simulink model "PitchPlunge"  (R2015a)
settings: Solver=ode3  StartTime=0.0  StopTime=T  FixedStep=dt  RelTol=1e-3
values from neighbouring files (symbols this model uses):
  dt = 0.01    [Main.m]
  gamma = 0.5    [Main.m]
  U0 = 15    [Main.m]
  useNonlinear = 0    [Main.m]
undefined symbols (not defined in the file or in its folder): C, D, E, F, initialTurbulence, ka, ka1, ka2, ka3, ka4, kh, Light, M, MIL, Q, R, stateFilterGamma, turbulenceFactor, turbulenceSeed, x0, xd0
libraries: aerolibwind2 x1
settings Model: Creator=hildobijl  LastModifiedBy=Hildo
settings DataIOCC: SignalLoggingSaveFormat=ModelDataLogs
settings OptimizationCC: ExpressionDepthLimit=2147483647
settings DebuggingCC: SolverPrmCheckMsg=warning  FcnCallInpInsideContextMsg=EnableAllAsWarning  StateNameClashWarn=warning
settings GRTTargetCC: CombineOutputUpdateFcns=off  GRTInterface=on

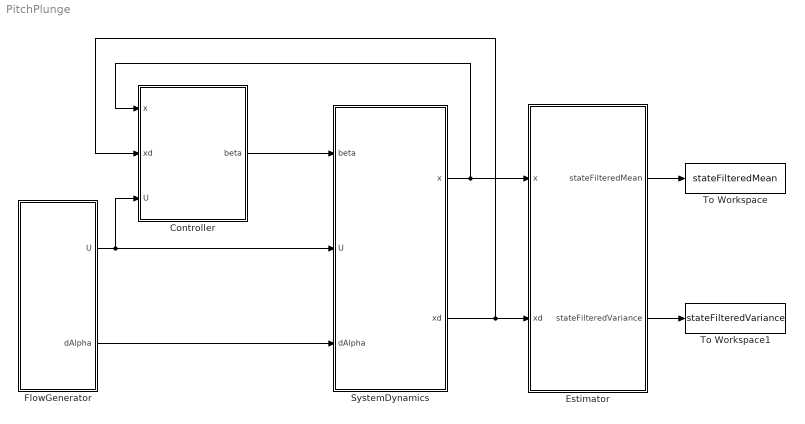
== system PitchPlunge ==
  Controller : Subsystem
  Estimator : Subsystem
  FlowGenerator : Subsystem
  SystemDynamics : Subsystem
  To Workspace : ToWorkspace  VariableName=stateFilteredMean  SampleTime=-1
  To Workspace1 : ToWorkspace  VariableName=stateFilteredVariance  SampleTime=-1
  wires:
  FlowGenerator/1(U) -> Controller/3(U), SystemDynamics/2(U)
  Controller/1(beta) -> SystemDynamics/1(beta)
  SystemDynamics/1(x) -> Controller/1(x), Estimator/1(x)
  SystemDynamics/2(xd) -> Controller/2(xd), Estimator/2(xd)
  FlowGenerator/2(dAlpha) -> SystemDynamics/3(dAlpha)
  Estimator/1(stateFilteredMean) -> To Workspace/1
  Estimator/2(stateFilteredVariance) -> To Workspace1/1

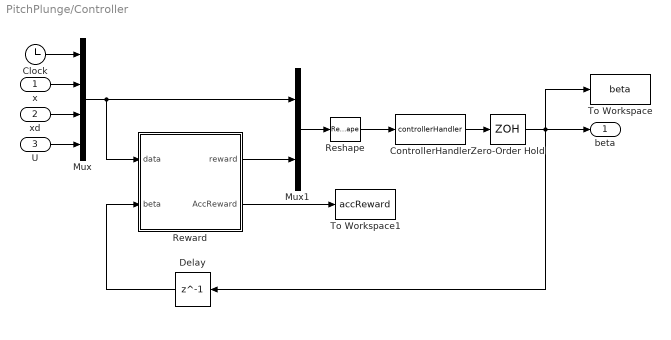
== system PitchPlunge/Controller ==
  x : Inport
  xd : Inport  Port=2
  U : Inport  Port=3
  Clock : Clock
  ControllerHandler : MATLABFcn  MATLABFcn=controllerHandler  SampleTime=dt
  Delay : Delay  DelayLength=1  InitialCondition=0
  Mux : Mux  Inputs=[1,2,2,1]
  Mux1 : Mux  Inputs=[6,1]
  Reshape : Reshape
  Reward : Subsystem
  To Workspace : ToWorkspace  VariableName=beta  SampleTime=-1
  To Workspace1 : ToWorkspace  VariableName=accReward  SampleTime=-1
  Zero-Order Hold : ZeroOrderHold  SampleTime=dt
  beta : Outport
  wires:
  Mux/1 -> Reward/1(data), Mux1/1
  Clock/1 -> Mux/1
  x/1 -> Mux/2
  xd/1 -> Mux/3
  U/1 -> Mux/4
  ControllerHandler/1 -> Zero-Order Hold/1
  Reward/1(reward) -> Mux1/2
  Mux1/1 -> Reshape/1
  Reshape/1 -> ControllerHandler/1
  Zero-Order Hold/1 -> Delay/1, beta/1, To Workspace/1
  Reward/2(AccReward) -> To Workspace1/1
  Delay/1 -> Reward/2(beta)

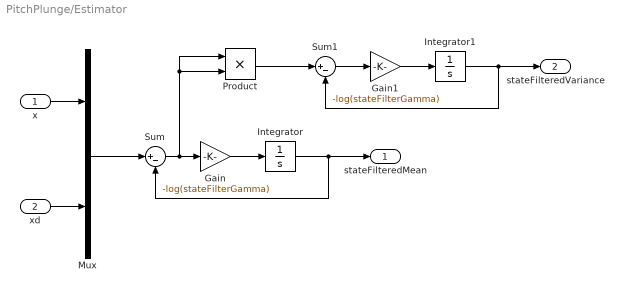
== system PitchPlunge/Estimator ==
  x : Inport
  xd : Inport  Port=2
  Gain : Gain  Gain=-log(stateFilterGamma)
  Gain1 : Gain  Gain=-log(stateFilterGamma)
  Integrator : Integrator  InitialCondition=[x0,xd0]'
  Integrator1 : Integrator
  Mux : Mux  Inputs=[2,2]
  Product : Product
  Sum : Sum  Inputs=|+-
  Sum1 : Sum  Inputs=|+-
  stateFilteredMean : Outport
  stateFilteredVariance : Outport  Port=2
  wires:
  x/1 -> Mux/1
  xd/1 -> Mux/2
  Mux/1 -> Sum/1
  Sum/1 -> Product/1, Product/2, Gain/1
  Integrator/1 -> Sum/2, stateFilteredMean/1
  Gain/1 -> Integrator/1
  Integrator1/1 -> Sum1/2, stateFilteredVariance/1
  Gain1/1 -> Integrator1/1
  Sum1/1 -> Gain1/1
  Product/1 -> Sum1/1

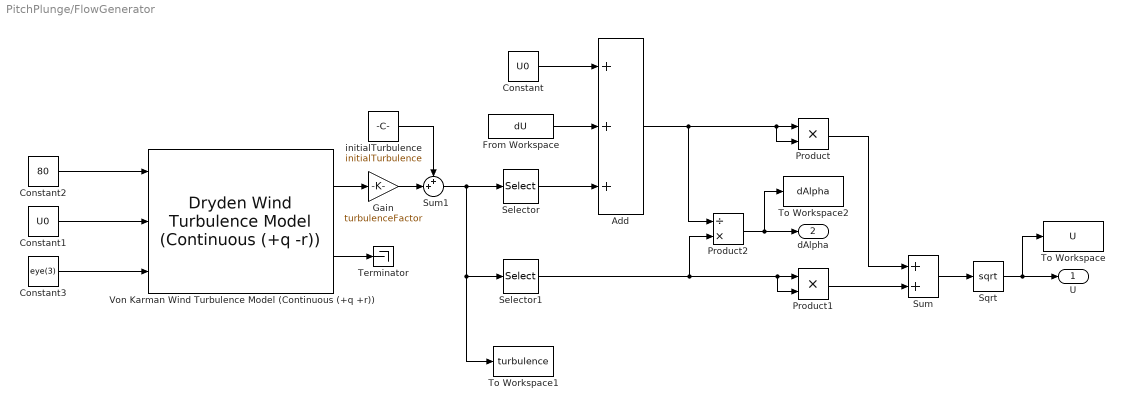
== system PitchPlunge/FlowGenerator ==
  Add : Sum  Inputs=+++
  Constant : Constant  Value=U0
  Constant1 : Constant  Value=U0
  Constant2 : Constant  Value=80
  Constant3 : Constant  Value=eye(3)
  From Workspace : FromWorkspace  VariableName=dU  SampleTime=dt  OutputAfterFinalValue=Holding final value
  Gain : Gain  Gain=turbulenceFactor
  Product : Product
  Product1 : Product
  Product2 : Product  Inputs=/*
  Selector : Selector  InputPortWidth=3  Indices=[1]
  Selector1 : Selector  InputPortWidth=3  Indices=[2]
  Sqrt : Sqrt  SaturateOnIntegerOverflow=on
  Sum : Sum
  Sum1 : Sum  Inputs=++|
  Terminator : Terminator
  To Workspace : ToWorkspace  VariableName=U  SampleTime=-1
  To Workspace1 : ToWorkspace  VariableName=turbulence  SampleTime=-1
  To Workspace2 : ToWorkspace  VariableName=dAlpha  SampleTime=-1
  Von Karman Wind Turbulence Model (Continuous (+q +r)) : aerolibwind2/Dryden Wind Turbulence Model  (Continuous (+q -r))  units=Metric (MKS)  spec=MIL-F-8785C  model=Continuous Von Karman (+q +r)  W20=U0  Wdeg=0  TurbProb=10^-2 - Light  L_high=762  Wingspan=10  ts=dt  Seed=turbulenceSeed  T_on=on
  initialTurbulence : Constant  Value=initialTurbulence
  U : Outport
  dAlpha : Outport  Port=2
  wires:
  Constant/1 -> Add/1
  From Workspace/1 -> Add/2
  Constant2/1 -> Von Karman Wind Turbulence Model (Continuous (+q +r))/1
  Constant1/1 -> Von Karman Wind Turbulence Model (Continuous (+q +r))/2
  Constant3/1 -> Von Karman Wind Turbulence Model (Continuous (+q +r))/3
  Von Karman Wind Turbulence Model (Continuous (+q +r))/2 -> Terminator/1
  Von Karman Wind Turbulence Model (Continuous (+q +r))/1 -> Gain/1
  Selector/1 -> Add/3
  Add/1 -> Product2/1, Product/2, Product/1
  Selector1/1 -> Product2/2, Product1/2, Product1/1
  Product/1 -> Sum/1
  Product1/1 -> Sum/2
  Sum/1 -> Sqrt/1
  Sqrt/1 -> U/1, To Workspace/1
  Product2/1 -> To Workspace2/1, dAlpha/1
  initialTurbulence/1 -> Sum1/1
  Gain/1 -> Sum1/2
  Sum1/1 -> To Workspace1/1, Selector1/1, Selector/1

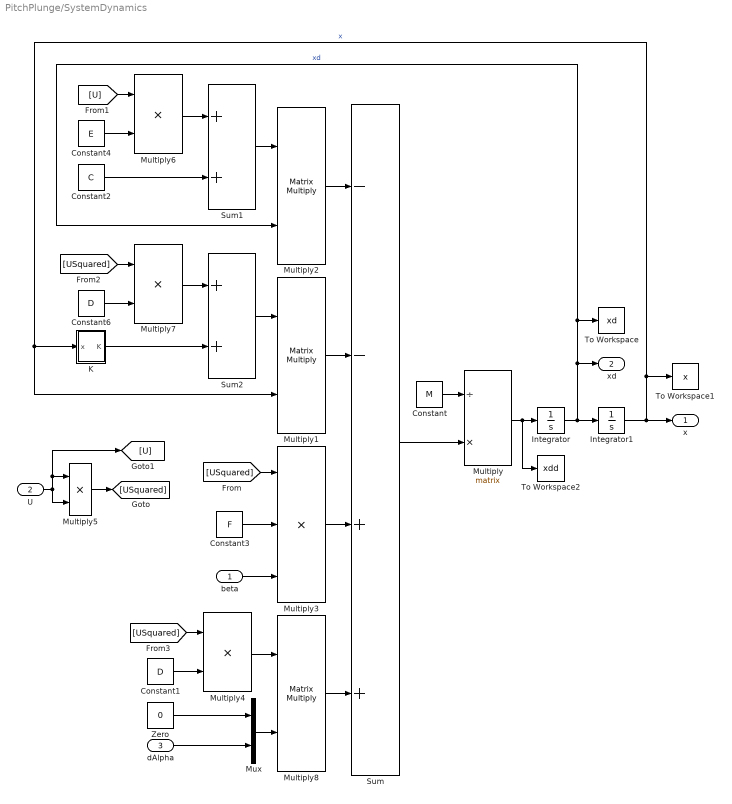
== system PitchPlunge/SystemDynamics ==
  beta : Inport
  U : Inport  Port=2
  dAlpha : Inport  Port=3
  Constant : Constant  Value=M
  Constant1 : Constant  Value=D
  Constant2 : Constant  Value=C
  Constant3 : Constant  Value=F
  Constant4 : Constant  Value=E
  Constant6 : Constant  Value=D
  Integrator : Integrator  InitialCondition=xd0
  Integrator1 : Integrator  InitialCondition=x0
  K : Subsystem
  Multiply : Product  Inputs=/*  Multiplication=Matrix(*)
  Multiply1 : Product  Inputs=**  Multiplication=Matrix(*)
  Multiply2 : Product  Inputs=**  Multiplication=Matrix(*)
  Multiply3 : Product  Inputs=***
  Multiply{4..7} (4 alike) : Product  Inputs=**
  Multiply8 : Product  Inputs=**  Multiplication=Matrix(*)
  Mux : Mux  Inputs=2
  Sum : Sum  Inputs=--++
  Sum1 : Sum
  Sum2 : Sum
  To Workspace : ToWorkspace  VariableName=xd  SampleTime=-1
  To Workspace1 : ToWorkspace  VariableName=x  SampleTime=-1
  To Workspace2 : ToWorkspace  VariableName=xdd  SampleTime=-1
  Zero : Constant  Value=0
  x : Outport
  xd : Outport  Port=2
  wires:
  Integrator/1 -> Integrator1/1, xd/1, To Workspace/1, Multiply2/2  "xd"
  Integrator1/1 -> x/1, To Workspace1/1, Multiply1/2, K/1(x)  "x"
  Multiply/1 -> To Workspace2/1, Integrator/1
  Constant/1 -> Multiply/1
  Sum/1 -> Multiply/2
  Multiply3/1 -> Sum/3
  Multiply2/1 -> Sum/1
  U/1 -> Multiply5/2, Multiply5/1, [U]
  Multiply5/1 -> [USquared]
  [U] -> Multiply6/1
  Constant4/1 -> Multiply6/2
  Multiply6/1 -> Sum1/1
  Constant2/1 -> Sum1/2
  Sum1/1 -> Multiply2/1
  [USquared] -> Multiply7/1
  Constant6/1 -> Multiply7/2
  Multiply7/1 -> Sum2/1
  Sum2/1 -> Multiply1/1
  Multiply1/1 -> Sum/2
  [USquared] -> Multiply3/1
  Constant3/1 -> Multiply3/2
  beta/1 -> Multiply3/3
  K/1(K) -> Sum2/2
  [USquared] -> Multiply4/1
  Constant1/1 -> Multiply4/2
  Zero/1 -> Mux/1
  dAlpha/1 -> Mux/2
  Multiply8/1 -> Sum/4
  Multiply4/1 -> Multiply8/1
  Mux/1 -> Multiply8/2

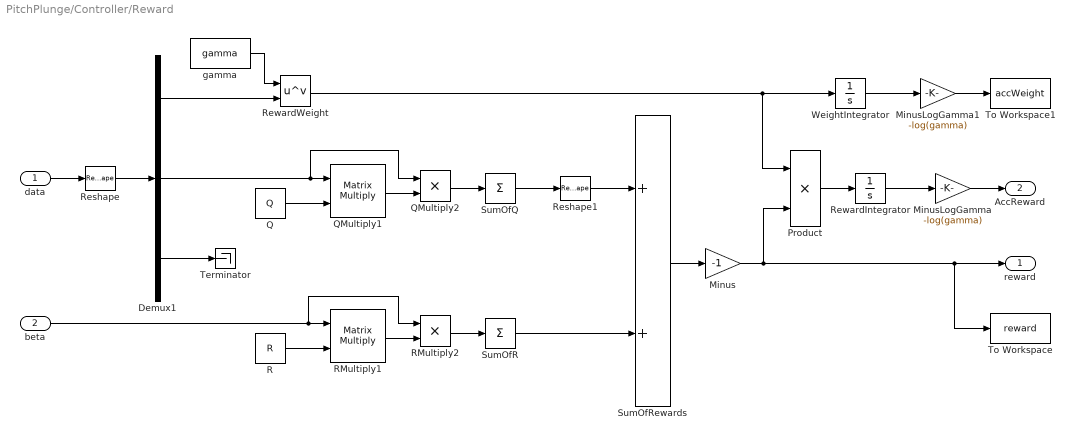
== system PitchPlunge/Controller/Reward ==
  data : Inport
  beta : Inport  Port=2
  Demux1 : Demux  Outputs=[1,4,1]
  Minus : Gain  Gain=-1
  MinusLogGamma : Gain  Gain=-log(gamma)
  MinusLogGamma1 : Gain  Gain=-log(gamma)
  Product : Product
  Q : Constant  Value=Q
  QMultiply1 : Product  Multiplication=Matrix(*)
  QMultiply2 : Product
  R : Constant  Value=R
  RMultiply1 : Product  Multiplication=Matrix(*)
  RMultiply2 : Product
  Reshape : Reshape
  Reshape1 : Reshape
  RewardIntegrator : Integrator
  RewardWeight : Math  Operator=pow  SaturateOnIntegerOverflow=on
  SumOfQ : Sum  Inputs=+
  SumOfR : Sum  Inputs=+
  SumOfRewards : Sum
  Terminator : Terminator
  To Workspace : ToWorkspace  VariableName=reward  SampleTime=-1
  To Workspace1 : ToWorkspace  VariableName=accWeight  SampleTime=-1
  WeightIntegrator : Integrator
  gamma : Constant  Value=gamma
  reward : Outport
  AccReward : Outport  Port=2
  wires:
  gamma/1 -> RewardWeight/1
  RewardWeight/1 -> WeightIntegrator/1, Product/1
  Product/1 -> RewardIntegrator/1
  RewardIntegrator/1 -> MinusLogGamma/1
  MinusLogGamma/1 -> AccReward/1
  WeightIntegrator/1 -> MinusLogGamma1/1
  MinusLogGamma1/1 -> To Workspace1/1
  Q/1 -> QMultiply1/2
  QMultiply1/1 -> QMultiply2/2
  QMultiply2/1 -> SumOfQ/1
  Demux1/2 -> QMultiply2/1, QMultiply1/1
  R/1 -> RMultiply1/2
  RMultiply1/1 -> RMultiply2/2
  RMultiply2/1 -> SumOfR/1
  SumOfR/1 -> SumOfRewards/2
  SumOfRewards/1 -> Minus/1
  beta/1 -> RMultiply2/1, RMultiply1/1
  Demux1/3 -> Terminator/1
  data/1 -> Reshape/1
  Reshape/1 -> Demux1/1
  SumOfQ/1 -> Reshape1/1
  Reshape1/1 -> SumOfRewards/1
  Demux1/1 -> RewardWeight/2
  Minus/1 -> reward/1, To Workspace/1, Product/2

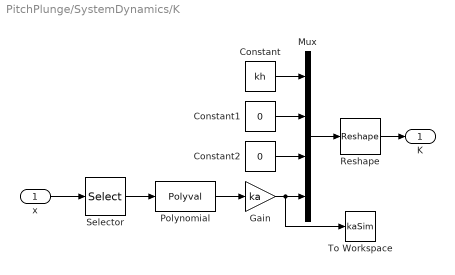
== system PitchPlunge/SystemDynamics/K ==
  x : Inport
  Constant : Constant  Value=kh
  Constant1 : Constant  Value=0
  Constant2 : Constant  Value=0
  Gain : Gain  Gain=ka
  Mux : Mux
  Polynomial : Polyval  Coefs=[useNonlinear*ka4,useNonlinear*ka3,useNonlinear*ka2,useNonlinear*ka1,1]
  Reshape : Reshape  OutputDimensionality=Customize  OutputDimensions=[2,2]
  Selector : Selector  InputPortWidth=2  Indices=[2]
  To Workspace : ToWorkspace  VariableName=kaSim  SampleTime=-1
  K : Outport
  wires:
  x/1 -> Selector/1
  Selector/1 -> Polynomial/1
  Polynomial/1 -> Gain/1
  Gain/1 -> Mux/4, To Workspace/1
  Mux/1 -> Reshape/1
  Reshape/1 -> K/1
  Constant/1 -> Mux/1
  Constant1/1 -> Mux/2
  Constant2/1 -> Mux/3
